simulink model "exampleStorage_type3"  (Simulink 8.2)
settings: Solver=ode45  StartTime=0.0  StopTime=3*3600-2  RelTol=1e-3
libraries: carnot x11, simulink x3
settings Model: Creator=drhf  LastModifiedBy=drhf

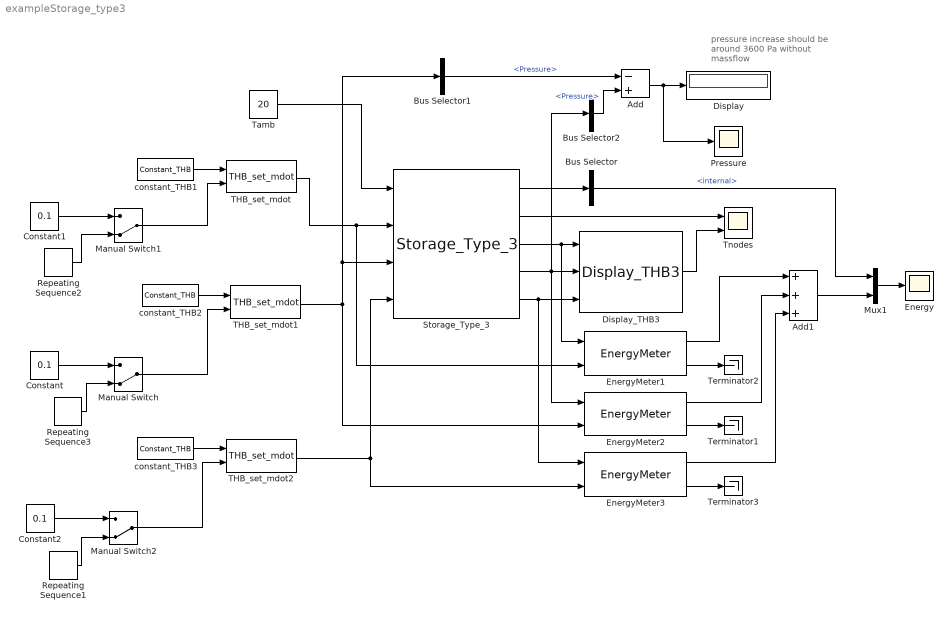
== system exampleStorage_type3 ==
  note: pressure increase should be around 3600 Pa without massflow
  Add : Sum  Inputs=-+
  Add1 : Sum  Inputs=3
  Bus Selector : BusSelector  OutputSignals=energy.internal
  Bus Selector1 : BusSelector  OutputSignals=Pressure
  Bus Selector2 : BusSelector  OutputSignals=Pressure
  Constant : Constant  Value=0.1
  Constant1 : Constant  Value=0.1
  Constant2 : Constant  Value=0.1
  Display : Display
  Display_THB3 : carnot/Outputs/Display_THB3  t=off  m=on  p=off  id=off  mix=off  d=off
  Energy : Scope
  EnergyMeter1 : carnot/Control/EnergyMeter
  EnergyMeter2 : carnot/Control/EnergyMeter
  EnergyMeter3 : carnot/Control/EnergyMeter
  Manual Switch : ManualSwitch  CurrentSetting=0
  Manual Switch1 : ManualSwitch  CurrentSetting=0
  Manual Switch2 : ManualSwitch  CurrentSetting=0
  Mux1 : Mux  Inputs=2
  Pressure : Scope
  Repeating Sequence1 : simulink/Sources/Repeating Sequence  rep_seq_t=[0 1 1.01 2 2.01 3]*3600  rep_seq_y=[0.12 0.12 0.11 0.11 0.05 0.05]
  Repeating Sequence2 : simulink/Sources/Repeating Sequence  rep_seq_t=[0 1 1.01 2 2.01 2.9 2.91 3.1]*3600  rep_seq_y=[0 0 0.05 0.05 0.2 0.2 0 0]
  Repeating Sequence3 : simulink/Sources/Repeating Sequence  rep_seq_t=[0 1 1.01 2 2.01 3]*3600  rep_seq_y=[0 0 0.1 0.1 0.15 0.15]
  Storage_Type_3 : carnot/Storage/Thermal/Storage_Type_3  uloss=1  ubot=1  utop=1  cond=1  t0=[10:5:55]  volume=0.3  dia=0.5  pos=standing cylinder  nconnect=3  nodes=10  mpoints=10
  THB_set_mdot : carnot/Source/Simple/THB_set_mdot
  THB_set_mdot1 : carnot/Source/Simple/THB_set_mdot
  THB_set_mdot2 : carnot/Source/Simple/THB_set_mdot
  Tamb : Constant  Value=20
  Terminator1 : Terminator
  Terminator2 : Terminator
  Terminator3 : Terminator
  Tnodes : Scope  NumInputPorts=2
      settings: YMin=-5~-5  YMax=5~5  SaveName=ScopeData3
  constant_THB1 : carnot/Source/Simple/Constant_THB  t=10  mdot=0*100/3600  p=1e5  mID=Full Pressure Drop with Static Height  fluid=Water  mix=0  dia=0.02  hgt=0
  constant_THB2 : carnot/Source/Simple/Constant_THB  t=55  mdot=0*100/3600  p=1e5  mID=Full Pressure Drop with Static Height  fluid=Water  mix=0  dia=0.02  hgt=0
  constant_THB3 : carnot/Source/Simple/Constant_THB  t=35  mdot=0*100/3600  p=1e5  mID=Full Pressure Drop with Static Height  fluid=Water  mix=0  dia=0.02  hgt=0
  wires:
  Bus Selector/1 -> Mux1/1  "<internal>"
  Tamb/1 -> Storage_Type_3/1
  THB_set_mdot/1 -> Storage_Type_3/2, EnergyMeter1/2
  THB_set_mdot1/1 -> Bus Selector1/1, Storage_Type_3/3, EnergyMeter2/2
  Storage_Type_3/1 -> Bus Selector/1
  Storage_Type_3/3 -> EnergyMeter1/1, Display_THB3/1
  Storage_Type_3/4 -> Bus Selector2/1, EnergyMeter2/1, Display_THB3/2
  Display_THB3/1 -> Tnodes/2
  Mux1/1 -> Energy/1
  EnergyMeter2/2 -> Terminator1/1
  Manual Switch1/1 -> THB_set_mdot/2
  Manual Switch/1 -> THB_set_mdot1/2
  Add/1 -> Display/1, Pressure/1
  Bus Selector1/1 -> Add/1  "<Pressure>"
  Bus Selector2/1 -> Add/2  "<Pressure>"
  Constant/1 -> Manual Switch/1
  Repeating Sequence3/1 -> Manual Switch/2
  Constant1/1 -> Manual Switch1/1
  Repeating Sequence2/1 -> Manual Switch1/2
  EnergyMeter1/2 -> Terminator2/1
  Add1/1 -> Mux1/2
  EnergyMeter2/1 -> Add1/2
  EnergyMeter1/1 -> Add1/1
  Manual Switch2/1 -> THB_set_mdot2/2
  Constant2/1 -> Manual Switch2/1
  Repeating Sequence1/1 -> Manual Switch2/2
  THB_set_mdot2/1 -> Storage_Type_3/4, EnergyMeter3/2
  Storage_Type_3/2 -> Tnodes/1
  Storage_Type_3/5 -> EnergyMeter3/1, Display_THB3/3
  EnergyMeter3/2 -> Terminator3/1
  EnergyMeter3/1 -> Add1/3
  constant_THB1/1 -> THB_set_mdot/1
  constant_THB2/1 -> THB_set_mdot1/1
  constant_THB3/1 -> THB_set_mdot2/1
